simulink model "MSD4Ways"  (R2021a)
settings: Solver=VariableStepAuto  StartTime=0.0  StopTime=10  FixedStep=0.01  RelTol=1e-3
PreLoadFcn:
  | k=30;
  | b=8;
  | m=5;
libraries: fl_lib x7, nesl_utility x3, sdl_lib x1
settings Model: Creator=rachelj  LastModifiedBy=smuckati
settings SolverCC: AlgebraicLoopSolver=TrustRegion
settings DebuggingCC: SFMachineParentedDataDiag=warning  ArithmeticOperatorsInVariantConditions=warning
settings SFSimCC: CustomCodeUndefinedFunction=UseInterfaceOnly

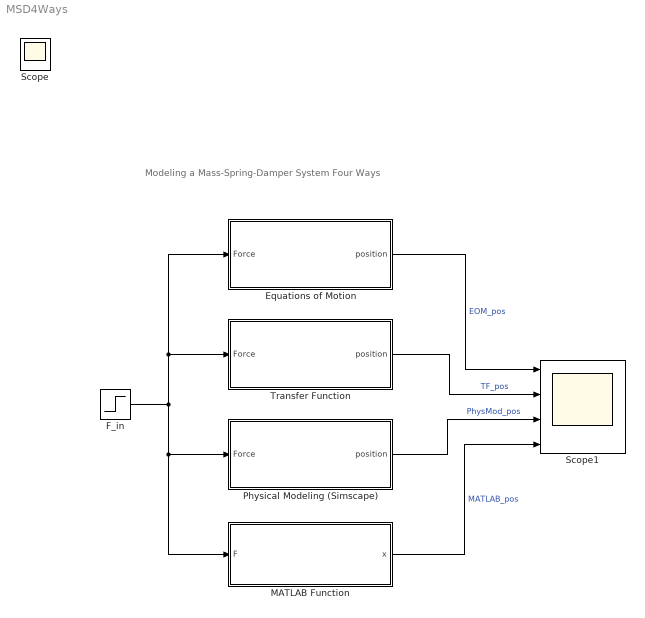
== system MSD4Ways ==
  note: Modeling a Mass-Spring-Damper System
      | Four Ways
  Equations of Motion : Subsystem
  F_in : Step  SampleTime=0
  MATLAB Function : MATLAB Function  TreatAsAtomicUnit=on
  Physical Modeling (Simscape) : Subsystem
  Scope1 : Scope  NumInputPorts=4
  Transfer Function : Subsystem
  Scope : Scope
  wires:
  Equations of Motion/1(" position") -> Scope1/1  "EOM_pos"
  Transfer Function/1(position) -> Scope1/2  "TF_pos"
  Physical Modeling (Simscape)/1(position) -> Scope1/3  "PhysMod_pos"
  F_in/1 -> Physical Modeling (Simscape)/1(Force), MATLAB Function/1(F), Equations of Motion/1(Force), Transfer Function/1(Force)
  MATLAB Function/1(x) -> Scope1/4  "MATLAB_pos"

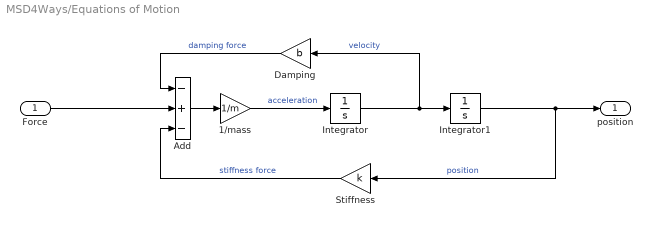
== system MSD4Ways/Equations of Motion ==
  Force : Inport
  1/mass : Gain  Gain=1/m
  Add : Sum  Inputs=-+-
  Damping : Gain  Gain=b
  Integrator : Integrator
  Integrator1 : Integrator
  Stiffness : Gain  Gain=k
  " position" : Outport  VectorParamsAs1DForOutWhenUnconnected=off
  wires:
  1/mass/1 -> Integrator/1  "acceleration"
  Damping/1 -> Add/1  "damping force"
  Integrator/1 -> Damping/1, Integrator1/1  "velocity"
  Force/1 -> Add/2
  Stiffness/1 -> Add/3  "stiffness force"
  Integrator1/1 -> " position"/1, Stiffness/1  "position"
  Add/1 -> 1/mass/1

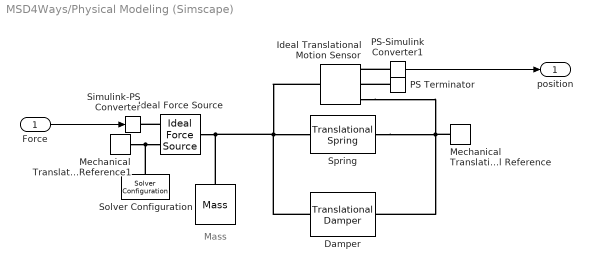
== system MSD4Ways/Physical Modeling (Simscape) ==
  note: Mass
  Force : Inport
  " " : fl_lib/Mechanical/Translational Elements/Mass  mass=m kg  num_ports=foundation.enum.numPorts2.one  v_specify=off  v_priority=High  v=0 m/s  v_nominal_specify=off  v_nominal_unit=m/s  v_nominal_value=1  f_specify=off  f_priority=None  f=0 N  f_nominal_specify=off  f_nominal_unit=N  f_nominal_value=1
  Damper : sdl_lib/Couplings & Drives/Springs & Dampers/Translational Damper  D=b N/(m/s)  enable_faults=0  b_fault=1e6 N/(m/s)  temporal_fault=0  fault_time=5 s  shock_fault=0  acceleration_limit=100 m/s^2  shock_limit=1  report_fault=1
      settings: SourceProductBaseCode=LD
  Ideal Force Source : fl_lib/Mechanical/Mechanical Sources/Ideal Force Source
  Ideal Translational Motion Sensor : fl_lib/Mechanical/Mechanical Sensors/Ideal Translational Motion Sensor  offset=0 m
  Mechanical Translational Reference : fl_lib/Mechanical/Translational Elements/Mechanical Translational Reference
  Mechanical Translational Reference1 : fl_lib/Mechanical/Translational Elements/Mechanical Translational Reference
  PS Terminator : fl_lib/Physical Signals/Sinks/PS Terminator
  PS-Simulink Converter1 : nesl_utility/PS-Simulink Converter  PhysicalDomain=network_engine_domain  SubClassName=ps_output  LeftPortType=input  RightPortType=output  PseudoPeriodic=off  Frequencies=[]  Unit=1  AffineConversion=off
      settings: SourceProductBaseCode=PW,SS
  Simulink-PS Converter : nesl_utility/Simulink-PS Converter  PhysicalDomain=network_engine_domain  SubClassName=ps_input  LeftPortType=input  RightPortType=output  PseudoPeriodic=off  Frequencies=[]  NoiseDistribution=none  NoiseParameters=[]  Unit=1  AffineConversion=off  FilteringAndDerivatives=provide  SimscapeFilterOrder=1  InputFilterTimeConstant=0.001  UdotUserProvided=0
      settings: SourceProductBaseCode=PW,SS
  Solver Configuration : nesl_utility/Solver Configuration  PhysicalDomain=network_engine_domain  SubClassName=solver  LeftPortType=input  RightPortType=generic  Tones=[]  Harmonics=[]  SimulateNoise=off  Profile=off  UseLocalSampling=off  EnableSwitchedLinearOptims=on  FrequencyDomain=off  UseCCode=off  RelTol=0.001  AbsTol=1e-06  MinStep=1e-09  ToWorkspace=off  RevertToSquareIcSolve=off  NumHomotopyIterations=100  PhasorMode=off  PhasorModeNumHarmonics=1  DoDC=off  ResidualTolerance=1e-09  UseLocalSolver=off  LocalSolverChoice=NE_BACKWARD_EULER_ADVANCER  LocalSolverSampleTime=0.001  DoFixedCost=off  MaxNonlinIter=3  MaxModeIter=2  ComputeImpulses=off  ImpulseIterations=2  LinearAlgebra=auto  EquationFormulation=NE_TIME_EF  DelaysMemoryBudget=1024  AutomaticFiltering=on  FilteringTimeConstant=0.001  PartitionStorageMethod=AS_NEEDED  PartitionMemoryBudget=1024  PartitionMethod=FAST
      settings: SourceProductBaseCode=PW,SS
  Spring : fl_lib/Mechanical/Translational Elements/Translational Spring  spr_rate=k N/m  v_specify=off  v_priority=None  v=0 m/s  v_nominal_specify=off  v_nominal_unit=m/s  v_nominal_value=1  f_specify=off  f_priority=None  f=0 N  f_nominal_specify=off  f_nominal_unit=N  f_nominal_value=1  x_specify=off  x_priority=High  x=0 m  x_nominal_specify=off  x_nominal_unit=m  x_nominal_value=1
  position : Outport  VectorParamsAs1DForOutWhenUnconnected=off
  wires:
  PS-Simulink Converter1/1 -> position/1
  Force/1 -> Simulink-PS Converter/1
  connections:
  PS-Simulink Converter1/LConn1 -- Ideal Translational Motion Sensor/RConn3
  Mechanical Translational Reference1/LConn1 -- Solver Configuration/RConn1 -- Ideal Force Source/RConn2
  Spring/RConn1 -- Mechanical Translational Reference/LConn1 -- Ideal Translational Motion Sensor/RConn1 -- Damper/RConn1
  Damper/LConn1 -- Spring/LConn1 -- Ideal Translational Motion Sensor/LConn1 -- Ideal Force Source/LConn1 -- " "/LConn1
  PS Terminator/LConn1 -- Ideal Translational Motion Sensor/RConn2
  Ideal Force Source/RConn1 -- Simulink-PS Converter/RConn1

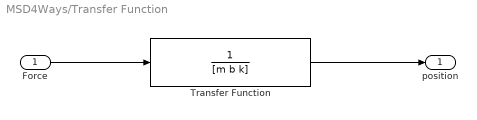
== system MSD4Ways/Transfer Function ==
  Force : Inport
  Transfer Function : TransferFcn  Denominator=[m b k]
  position : Outport  VectorParamsAs1DForOutWhenUnconnected=off
  wires:
  Force/1 -> Transfer Function/1
  Transfer Function/1 -> position/1

== matlab function MSD4Ways/MATLAB Function ==
  settings: updateMethod=DISCRETE  sampleTime=0.01
  data: F input; x output; k parameter; m parameter; b parameter
%% MSD MATLAB Function
% Updates the position x of a mass-spring-damper system with parameters k,
% b, and m based on an input force F

function x = msd(F,k,m,b)

persistent xprev vprev

% timestep must be identical to discrete rate in Simulink 
deltaT = 0.01;

% initialize for first timestep
if isempty(xprev)
    xprev = 0;
    vprev = 0;
end
    
    % calculate acceleration from previous position and velocity values
    a = (F - b*vprev - k*xprev)/m;
    
    % update velocity
    v = a*deltaT + vprev;

    % update position
    x = v*deltaT + xprev;

    % set velocity and position for next timestep
    vprev = v;
    xprev = x;
